simulink model "lab4_test2"  (R2016b)
settings: Solver=VariableStepAuto  StartTime=0.0  StopTime=totaltime  RelTol=1e-3
undefined symbols (not defined in the file or in its folder): h, st
libraries: xbsIndex_r4 x885
(part 1 of 2)
settings Model: Creator=rm101  LastModifiedBy=rm101

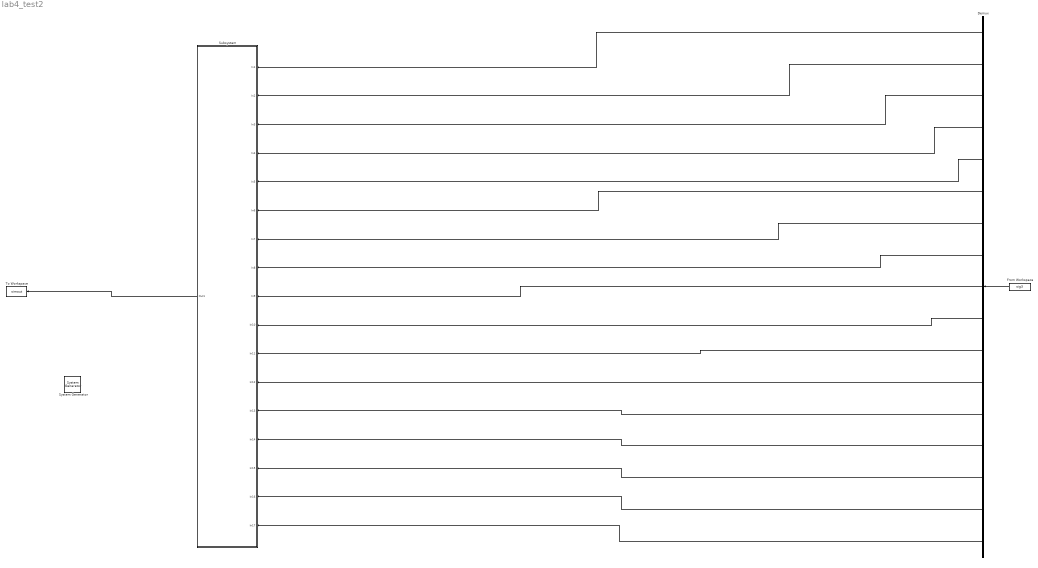
== system lab4_test2 ==
  " System Generator" : xbsIndex_r4/ System Generator  Tag=genX  xilinxfamily=zynq  part=xc7z020  speed=-1  package=clg484  synthesis_tool=Vivado  clock_wrapper=Clock Enables  directory=C:/Users/rm101/Desktop/YG/Lab4_Matlab/gen  proj_type=Vivado  Synth_file=Vivado Synthesis Defaults  Impl_file=Vivado Implementation Defaults  testbench=off  simulink_period=st  sysclk_period=st*10e8  dcm_input_clock_period=10  incr_netlist=off  trim_vbits=Everywhere in SubSystem  dbl_ovrd=According to Block Masks  core_generation=According to Block Masks  run_coregen=off  deprecated_control=off  eval_field=0  block_type=sysgen
  Demux : Demux  Outputs=17
  From Workspace : FromWorkspace  VariableName=sig3  SampleTime=0  Interpolate=off  OutputAfterFinalValue=Holding final value
  Subsystem : Subsystem
  To Workspace : ToWorkspace  VariableName=simout  SaveFormat=Timeseries  SampleTime=-1
  wires:
  From Workspace/1 -> Demux/1
  Demux/1 -> Subsystem/1(In1)
  Demux/2 -> Subsystem/2(In2)
  Demux/3 -> Subsystem/3(In3)
  Demux/4 -> Subsystem/4(In4)
  Demux/5 -> Subsystem/5(In5)
  Demux/6 -> Subsystem/6(In6)
  Demux/7 -> Subsystem/7(In7)
  Demux/8 -> Subsystem/8(In8)
  Demux/9 -> Subsystem/9(In9)
  Demux/10 -> Subsystem/10(In10)
  Demux/11 -> Subsystem/11(In11)
  Demux/12 -> Subsystem/12(In12)
  Demux/13 -> Subsystem/13(In13)
  Demux/14 -> Subsystem/14(In14)
  Demux/15 -> Subsystem/15(In15)
  Demux/16 -> Subsystem/16(In16)
  Demux/17 -> Subsystem/17(In17)
  Subsystem/1(Out1) -> To Workspace/1

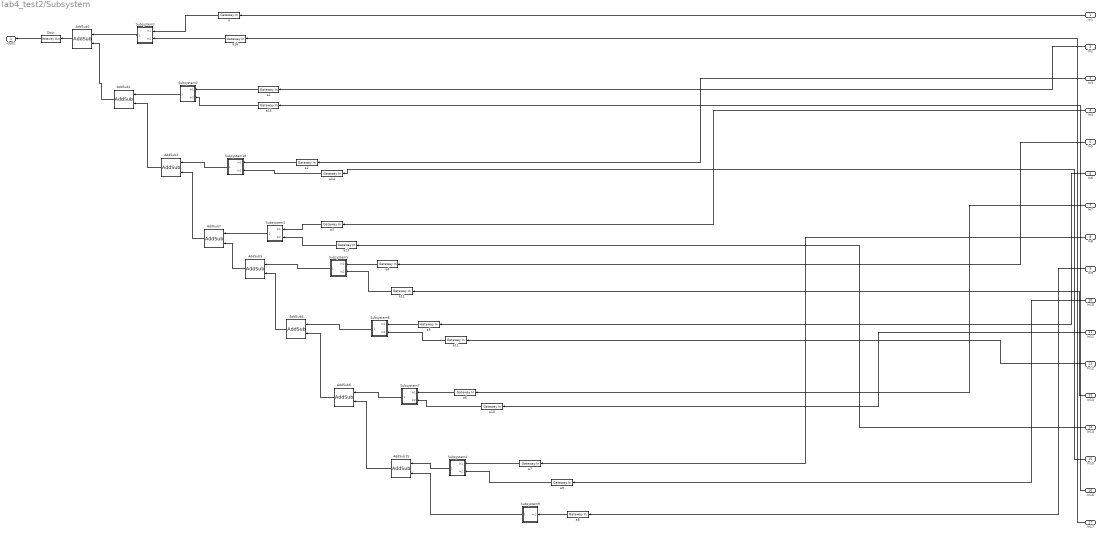
== system lab4_test2/Subsystem ==
  In1 : Inport
  In2 : Inport  Port=2
  In3 : Inport  Port=3
  In4 : Inport  Port=4
  In5 : Inport  Port=5
  In6 : Inport  Port=6
  In7 : Inport  Port=7
  In8 : Inport  Port=8
  In9 : Inport  Port=9
  In10 : Inport  Port=10
  In11 : Inport  Port=11
  In12 : Inport  Port=12
  In13 : Inport  Port=13
  In14 : Inport  Port=14
  In15 : Inport  Port=15
  In16 : Inport  Port=16
  In17 : Inport  Port=17
  AddSub{1..7,15} (8 alike) : xbsIndex_r4/AddSub  mode=Addition  use_carryin=off  use_carryout=off  en=off  latency=0  precision=User Defined  arith_type="Signed  (2's comp)"  n_bits=17  bin_pt=14  quantization=Truncate  overflow=Wrap  use_behavioral_HDL=off  hw_selection=Fabric  pipelined=off  dbl_ovrd=off  block_type=addsub
  Dout : xbsIndex_r4/Gateway Out  inherit_from_input=off  hdl_port=on  rows=1  columns=1  UseAsDAC=off  DACChannel='1'  interface=None  automatic_assignment=on  address_offset=hex2dec('00')  intf_name=''  intf_description=''  timing_constraint=None  locs_specified=off  LOCs={}  io_standard={}  block_type=gatewayout
  Subsystem1 : Subsystem
  Subsystem18 : Subsystem
  Subsystem2 : Subsystem
  Subsystem3 : Subsystem
  Subsystem4 : Subsystem
  Subsystem5 : Subsystem
  Subsystem6 : Subsystem
  Subsystem7 : Subsystem
  Subsystem9 : Subsystem
  a{,1..16} (17 alike) : xbsIndex_r4/Gateway In  gui_display_data_type=Fixed-point  arith_type="Signed  (2's comp)"  n_bits=8  bin_pt=6  preci_type=Single  exp_width=8  frac_width=24  rows=1  columns=1  quantization="Round  (unbiased: +/- Inf)"  overflow=Saturate  period=st  UseAsADC=off  ADCChannel='1'  interface=None  automatic_assignment=on  address_offset=hex2dec('00')  intf_name=''  intf_description=''  default_value=0  timing_constraint=None  locs_specified=off  LOCs={}  io_standard={}  inherit_from_input=off  hdl_port=on  dbl_ovrd=off  block_type=gatewayin
  Out1 : Outport
  wires:
  a10/1 -> Subsystem7/2(In2)
  a12/1 -> Subsystem5/2(In2)
  a11/1 -> Subsystem6/2(In2)
  a13/1 -> Subsystem3/2(In2)
  a9/1 -> Subsystem4/2(In2)
  Dout/1 -> Out1/1
  AddSub2/1 -> Dout/1
  Subsystem1/1(Out1) -> AddSub2/1
  AddSub1/1 -> AddSub2/2
  Subsystem2/1(Out1) -> AddSub1/1
  AddSub3/1 -> AddSub1/2
  Subsystem18/1(Out1) -> AddSub3/1
  AddSub7/1 -> AddSub3/2
  AddSub5/1 -> AddSub7/2
  Subsystem5/1(Out1) -> AddSub5/1
  AddSub4/1 -> AddSub5/2
  Subsystem6/1(Out1) -> AddSub4/1
  AddSub6/1 -> AddSub4/2
  Subsystem7/1(Out1) -> AddSub6/1
  AddSub15/1 -> AddSub6/2
  Subsystem3/1(Out1) -> AddSub7/1
  Subsystem4/1(Out1) -> AddSub15/1
  Subsystem9/1(Out1) -> AddSub15/2
  In2/1 -> a1/1
  In3/1 -> a2/1
  In4/1 -> a3/1
  In5/1 -> a4/1
  In6/1 -> a5/1
  In7/1 -> a6/1
  In8/1 -> a7/1
  In9/1 -> a8/1
  In10/1 -> a9/1
  In11/1 -> a10/1
  In12/1 -> a11/1
  In13/1 -> a12/1
  In14/1 -> a13/1
  In15/1 -> a14/1
  In16/1 -> a15/1
  In17/1 -> a16/1
  In1/1 -> a/1
  a/1 -> Subsystem1/1(In1)
  a1/1 -> Subsystem2/1(In1)
  a3/1 -> Subsystem3/1(In1)
  a2/1 -> Subsystem18/1(In1)
  a4/1 -> Subsystem5/1(In1)
  a5/1 -> Subsystem6/1(In1)
  a6/1 -> Subsystem7/1(In1)
  a7/1 -> Subsystem4/1(In1)
  a8/1 -> Subsystem9/1(In1)
  a14/1 -> Subsystem18/2(In2)
  a16/1 -> Subsystem1/2(In2)
  a15/1 -> Subsystem2/2(In2)

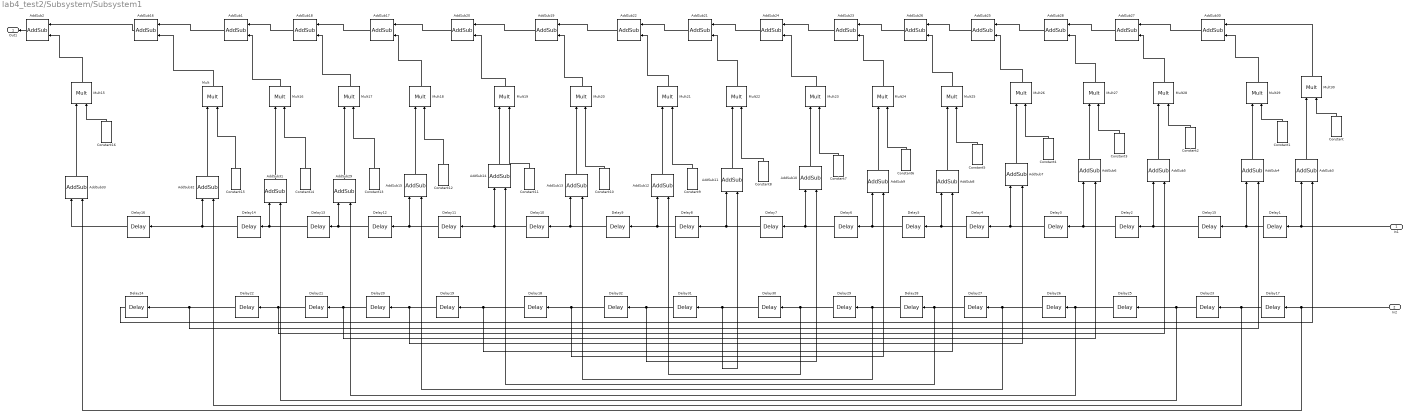
== system lab4_test2/Subsystem/Subsystem1 ==
  In1 : Inport
  In2 : Inport  Port=2
  AddSub{1..33} (33 alike) : xbsIndex_r4/AddSub  mode=Addition  use_carryin=off  use_carryout=off  en=off  latency=0  precision=User Defined  arith_type="Signed  (2's comp)"  n_bits=W  bin_pt=B  quantization=Truncate  overflow=Wrap  use_behavioral_HDL=off  hw_selection=Fabric  pipelined=off  dbl_ovrd=off  block_type=addsub
  Constant : xbsIndex_r4/Constant  const=h(1,17)  gui_display_data_type=Fixed-point  arith_type=Signed (2's comp)  n_bits=W  bin_pt=B  preci_type=Single  exp_width=8  frac_width=24  explicit_period=off  period=1  equ=P=C  opselect=C  inp2=PCIN>>17  opr=+  inp1=P  carry=CIN  dbl_ovrd=off  block_type=constant
  Constant1 : xbsIndex_r4/Constant  const=h(2,17)  gui_display_data_type=Fixed-point  arith_type=Signed (2's comp)  n_bits=W  bin_pt=B  preci_type=Single  exp_width=8  frac_width=24  explicit_period=off  period=1  equ=P=C  opselect=C  inp2=PCIN>>17  opr=+  inp1=P  carry=CIN  dbl_ovrd=off  block_type=constant
  Constant10 : xbsIndex_r4/Constant  const=h(11,17)  gui_display_data_type=Fixed-point  arith_type=Signed (2's comp)  n_bits=W  bin_pt=B  preci_type=Single  exp_width=8  frac_width=24  explicit_period=off  period=1  equ=P=C  opselect=C  inp2=PCIN>>17  opr=+  inp1=P  carry=CIN  dbl_ovrd=off  block_type=constant
  Constant11 : xbsIndex_r4/Constant  const=h(12,17)  gui_display_data_type=Fixed-point  arith_type=Signed (2's comp)  n_bits=W  bin_pt=B  preci_type=Single  exp_width=8  frac_width=24  explicit_period=off  period=1  equ=P=C  opselect=C  inp2=PCIN>>17  opr=+  inp1=P  carry=CIN  dbl_ovrd=off  block_type=constant
  Constant12 : xbsIndex_r4/Constant  const=h(13,17)  gui_display_data_type=Fixed-point  arith_type=Signed (2's comp)  n_bits=W  bin_pt=B  preci_type=Single  exp_width=8  frac_width=24  explicit_period=off  period=1  equ=P=C  opselect=C  inp2=PCIN>>17  opr=+  inp1=P  carry=CIN  dbl_ovrd=off  block_type=constant
  Constant13 : xbsIndex_r4/Constant  const=h(14,17)  gui_display_data_type=Fixed-point  arith_type=Signed (2's comp)  n_bits=W  bin_pt=B  preci_type=Single  exp_width=8  frac_width=24  explicit_period=off  period=1  equ=P=C  opselect=C  inp2=PCIN>>17  opr=+  inp1=P  carry=CIN  dbl_ovrd=off  block_type=constant
  Constant14 : xbsIndex_r4/Constant  const=h(15,17)  gui_display_data_type=Fixed-point  arith_type=Signed (2's comp)  n_bits=W  bin_pt=B  preci_type=Single  exp_width=8  frac_width=24  explicit_period=off  period=1  equ=P=C  opselect=C  inp2=PCIN>>17  opr=+  inp1=P  carry=CIN  dbl_ovrd=off  block_type=constant
  Constant15 : xbsIndex_r4/Constant  const=h(16,17)  gui_display_data_type=Fixed-point  arith_type=Signed (2's comp)  n_bits=W  bin_pt=B  preci_type=Single  exp_width=8  frac_width=24  explicit_period=off  period=1  equ=P=C  opselect=C  inp2=PCIN>>17  opr=+  inp1=P  carry=CIN  dbl_ovrd=off  block_type=constant
  Constant16 : xbsIndex_r4/Constant  const=h(17,17)  gui_display_data_type=Fixed-point  arith_type=Signed (2's comp)  n_bits=W  bin_pt=B  preci_type=Single  exp_width=8  frac_width=24  explicit_period=off  period=1  equ=P=C  opselect=C  inp2=PCIN>>17  opr=+  inp1=P  carry=CIN  dbl_ovrd=off  block_type=constant
  Constant2 : xbsIndex_r4/Constant  const=h(3,17)  gui_display_data_type=Fixed-point  arith_type=Signed (2's comp)  n_bits=W  bin_pt=B  preci_type=Single  exp_width=8  frac_width=24  explicit_period=off  period=1  equ=P=C  opselect=C  inp2=PCIN>>17  opr=+  inp1=P  carry=CIN  dbl_ovrd=off  block_type=constant
  Constant3 : xbsIndex_r4/Constant  const=h(4,17)  gui_display_data_type=Fixed-point  arith_type=Signed (2's comp)  n_bits=W  bin_pt=B  preci_type=Single  exp_width=8  frac_width=24  explicit_period=off  period=1  equ=P=C  opselect=C  inp2=PCIN>>17  opr=+  inp1=P  carry=CIN  dbl_ovrd=off  block_type=constant
  Constant4 : xbsIndex_r4/Constant  const=h(5,17)  gui_display_data_type=Fixed-point  arith_type=Signed (2's comp)  n_bits=W  bin_pt=B  preci_type=Single  exp_width=8  frac_width=24  explicit_period=off  period=1  equ=P=C  opselect=C  inp2=PCIN>>17  opr=+  inp1=P  carry=CIN  dbl_ovrd=off  block_type=constant
  Constant5 : xbsIndex_r4/Constant  const=h(6,17)  gui_display_data_type=Fixed-point  arith_type=Signed (2's comp)  n_bits=W  bin_pt=B  preci_type=Single  exp_width=8  frac_width=24  explicit_period=off  period=1  equ=P=C  opselect=C  inp2=PCIN>>17  opr=+  inp1=P  carry=CIN  dbl_ovrd=off  block_type=constant
  Constant6 : xbsIndex_r4/Constant  const=h(7,17)  gui_display_data_type=Fixed-point  arith_type=Signed (2's comp)  n_bits=W  bin_pt=B  preci_type=Single  exp_width=8  frac_width=24  explicit_period=off  period=1  equ=P=C  opselect=C  inp2=PCIN>>17  opr=+  inp1=P  carry=CIN  dbl_ovrd=off  block_type=constant
  Constant7 : xbsIndex_r4/Constant  const=h(8,17)  gui_display_data_type=Fixed-point  arith_type=Signed (2's comp)  n_bits=W  bin_pt=B  preci_type=Single  exp_width=8  frac_width=24  explicit_period=off  period=1  equ=P=C  opselect=C  inp2=PCIN>>17  opr=+  inp1=P  carry=CIN  dbl_ovrd=off  block_type=constant
  Constant8 : xbsIndex_r4/Constant  const=h(9,17)  gui_display_data_type=Fixed-point  arith_type=Signed (2's comp)  n_bits=W  bin_pt=B  preci_type=Single  exp_width=8  frac_width=24  explicit_period=off  period=1  equ=P=C  opselect=C  inp2=PCIN>>17  opr=+  inp1=P  carry=CIN  dbl_ovrd=off  block_type=constant
  Constant9 : xbsIndex_r4/Constant  const=h(10,17)  gui_display_data_type=Fixed-point  arith_type=Signed (2's comp)  n_bits=W  bin_pt=B  preci_type=Single  exp_width=8  frac_width=24  explicit_period=off  period=1  equ=P=C  opselect=C  inp2=PCIN>>17  opr=+  inp1=P  carry=CIN  dbl_ovrd=off  block_type=constant
  Delay{1..32} (32 alike) : xbsIndex_r4/Delay  rst=off  infoeditControl=Selection of Reset will increase slice count due to use of real FFs and instead of SRLs  en=off  latency=1  reg_retiming=off  dbl_ovrd=off  block_type=delay
  Mult{,15..30} (17 alike) : xbsIndex_r4/Mult  precision=User Defined  arith_type="Signed  (2's comp)"  n_bits=W  bin_pt=B  quantization="Round  (unbiased: +/- Inf)"  overflow=Flag as error  en=off  latency=0  use_behavioral_HDL=off  opt=Speed  use_embedded=on  optimum_pipeline=off  pipeline=on  dbl_ovrd=off  use_rpm=on  placement_style=Triangular  block_type=mult
  Out1 : Outport
  wires:
  AddSub2/1 -> Out1/1
  Constant14/1 -> Mult16/2
  Mult/1 -> AddSub16/2
  Mult16/1 -> AddSub1/2
  Constant15/1 -> Mult/2
  Constant13/1 -> Mult17/2
  Mult17/1 -> AddSub18/2
  Constant12/1 -> Mult18/2
  Constant11/1 -> Mult19/2
  Mult19/1 -> AddSub20/2
  Constant10/1 -> Mult20/2
  Mult20/1 -> AddSub19/2
  Constant9/1 -> Mult21/2
  Mult21/1 -> AddSub22/2
  Constant8/1 -> Mult22/2
  Constant7/1 -> Mult23/2
  Mult23/1 -> AddSub24/2
  Constant6/1 -> Mult24/2
  Constant5/1 -> Mult25/2
  Mult25/1 -> AddSub26/2
  Constant4/1 -> Mult26/2
  Mult26/1 -> AddSub25/2
  Constant3/1 -> Mult27/2
  Mult27/1 -> AddSub28/2
  Constant2/1 -> Mult28/2
  Constant1/1 -> Mult29/2
  Mult29/1 -> AddSub30/2
  Constant/1 -> Mult30/2
  AddSub1/1 -> AddSub16/1
  AddSub18/1 -> AddSub1/1
  AddSub17/1 -> AddSub18/1
  AddSub19/1 -> AddSub20/1
  AddSub22/1 -> AddSub19/1
  AddSub21/1 -> AddSub22/1
  AddSub23/1 -> AddSub24/1
  AddSub25/1 -> AddSub26/1
  AddSub28/1 -> AddSub25/1
  AddSub27/1 -> AddSub28/1
  Mult30/1 -> AddSub30/1
  Constant16/1 -> Mult15/2
  Mult15/1 -> AddSub2/2
  AddSub16/1 -> AddSub2/1
  AddSub20/1 -> AddSub17/1
  Mult18/1 -> AddSub17/2
  AddSub24/1 -> AddSub21/1
  Mult22/1 -> AddSub21/2
  AddSub26/1 -> AddSub23/1
  Mult24/1 -> AddSub23/2
  AddSub30/1 -> AddSub27/1
  Mult28/1 -> AddSub27/2
  In1/1 -> AddSub3/1, Delay1/1
  Delay1/1 -> AddSub4/1, Delay15/1
  Delay15/1 -> AddSub5/1, Delay2/1
  Delay2/1 -> AddSub6/1, Delay3/1
  Delay3/1 -> AddSub7/1, Delay4/1
  Delay4/1 -> AddSub8/1, Delay5/1
  Delay5/1 -> AddSub9/1, Delay6/1
  Delay6/1 -> AddSub10/1, Delay7/1
  Delay7/1 -> AddSub11/1, Delay8/1
  Delay8/1 -> AddSub12/1, Delay9/1
  Delay9/1 -> AddSub13/1, Delay10/1
  Delay10/1 -> AddSub14/1, Delay11/1
  Delay11/1 -> AddSub15/1, Delay12/1
  Delay12/1 -> AddSub29/1, Delay13/1
  Delay13/1 -> AddSub31/1, Delay14/1
  Delay14/1 -> AddSub32/1, Delay16/1
  In2/1 -> AddSub33/2, Delay17/1
  Delay17/1 -> AddSub32/2, Delay23/1
  Delay23/1 -> AddSub31/2, Delay25/1
  Delay25/1 -> AddSub29/2, Delay26/1
  Delay26/1 -> AddSub15/2, Delay27/1
  Delay27/1 -> AddSub14/2, Delay28/1
  Delay28/1 -> AddSub13/2, Delay29/1
  Delay29/1 -> AddSub12/2, Delay30/1
  Delay30/1 -> AddSub11/2, Delay31/1
  Delay31/1 -> AddSub10/2, Delay32/1
  Delay32/1 -> AddSub9/2, Delay18/1
  Delay18/1 -> AddSub8/2, Delay19/1
  Delay19/1 -> AddSub7/2, Delay20/1
  Delay20/1 -> AddSub6/2, Delay21/1
  Delay21/1 -> AddSub5/2, Delay22/1
  Delay22/1 -> AddSub4/2, Delay24/1
  AddSub3/1 -> Mult30/1
  Delay16/1 -> AddSub33/1
  AddSub33/1 -> Mult15/1
  AddSub32/1 -> Mult/1
  AddSub31/1 -> Mult16/1
  AddSub29/1 -> Mult17/1
  AddSub15/1 -> Mult18/1
  AddSub14/1 -> Mult19/1
  AddSub13/1 -> Mult20/1
  AddSub12/1 -> Mult21/1
  AddSub11/1 -> Mult22/1
  AddSub10/1 -> Mult23/1
  AddSub9/1 -> Mult24/1
  AddSub8/1 -> Mult25/1
  AddSub7/1 -> Mult26/1
  AddSub6/1 -> Mult27/1
  AddSub5/1 -> Mult28/1
  AddSub4/1 -> Mult29/1
  Delay24/1 -> AddSub3/2

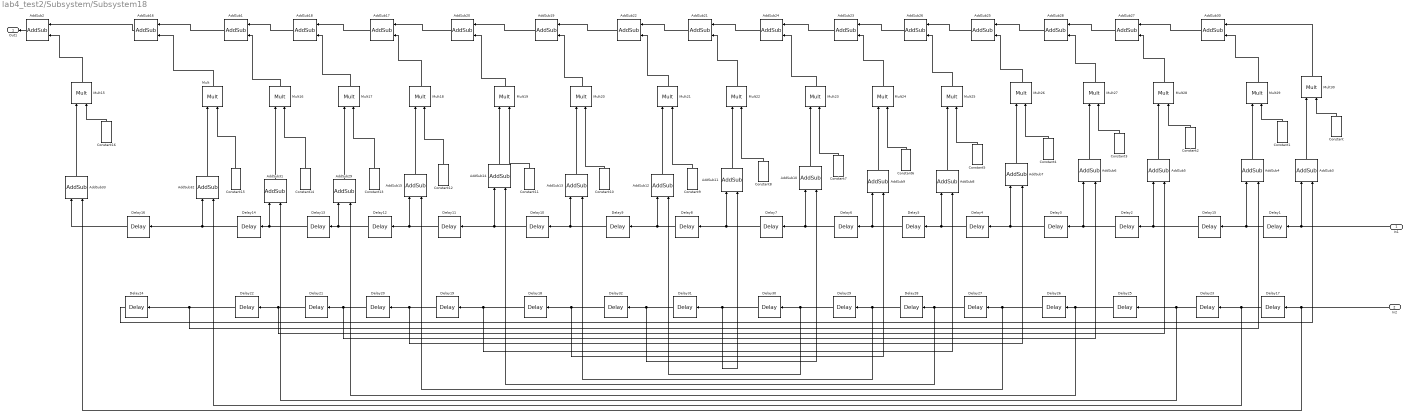
== system lab4_test2/Subsystem/Subsystem18 ==
  In1 : Inport
  In2 : Inport  Port=2
  AddSub{1..33} (33 alike) : xbsIndex_r4/AddSub  mode=Addition  use_carryin=off  use_carryout=off  en=off  latency=0  precision=User Defined  arith_type="Signed  (2's comp)"  n_bits=W  bin_pt=B  quantization=Truncate  overflow=Wrap  use_behavioral_HDL=off  hw_selection=Fabric  pipelined=off  dbl_ovrd=off  block_type=addsub
  Constant : xbsIndex_r4/Constant  const=h(1,15)  gui_display_data_type=Fixed-point  arith_type=Signed (2's comp)  n_bits=W  bin_pt=B  preci_type=Single  exp_width=8  frac_width=24  explicit_period=off  period=1  equ=P=C  opselect=C  inp2=PCIN>>17  opr=+  inp1=P  carry=CIN  dbl_ovrd=off  block_type=constant
  Constant1 : xbsIndex_r4/Constant  const=h(2,15)  gui_display_data_type=Fixed-point  arith_type=Signed (2's comp)  n_bits=W  bin_pt=B  preci_type=Single  exp_width=8  frac_width=24  explicit_period=off  period=1  equ=P=C  opselect=C  inp2=PCIN>>17  opr=+  inp1=P  carry=CIN  dbl_ovrd=off  block_type=constant
  Constant10 : xbsIndex_r4/Constant  const=h(11,15)  gui_display_data_type=Fixed-point  arith_type=Signed (2's comp)  n_bits=W  bin_pt=B  preci_type=Single  exp_width=8  frac_width=24  explicit_period=off  period=1  equ=P=C  opselect=C  inp2=PCIN>>17  opr=+  inp1=P  carry=CIN  dbl_ovrd=off  block_type=constant
  Constant11 : xbsIndex_r4/Constant  const=h(12,15)  gui_display_data_type=Fixed-point  arith_type=Signed (2's comp)  n_bits=W  bin_pt=B  preci_type=Single  exp_width=8  frac_width=24  explicit_period=off  period=1  equ=P=C  opselect=C  inp2=PCIN>>17  opr=+  inp1=P  carry=CIN  dbl_ovrd=off  block_type=constant
  Constant12 : xbsIndex_r4/Constant  const=h(13,15)  gui_display_data_type=Fixed-point  arith_type=Signed (2's comp)  n_bits=W  bin_pt=B  preci_type=Single  exp_width=8  frac_width=24  explicit_period=off  period=1  equ=P=C  opselect=C  inp2=PCIN>>17  opr=+  inp1=P  carry=CIN  dbl_ovrd=off  block_type=constant
  Constant13 : xbsIndex_r4/Constant  const=h(14,15)  gui_display_data_type=Fixed-point  arith_type=Signed (2's comp)  n_bits=W  bin_pt=B  preci_type=Single  exp_width=8  frac_width=24  explicit_period=off  period=1  equ=P=C  opselect=C  inp2=PCIN>>17  opr=+  inp1=P  carry=CIN  dbl_ovrd=off  block_type=constant
  Constant14 : xbsIndex_r4/Constant  const=h(15,15)  gui_display_data_type=Fixed-point  arith_type=Signed (2's comp)  n_bits=W  bin_pt=B  preci_type=Single  exp_width=8  frac_width=24  explicit_period=off  period=1  equ=P=C  opselect=C  inp2=PCIN>>17  opr=+  inp1=P  carry=CIN  dbl_ovrd=off  block_type=constant
  Constant15 : xbsIndex_r4/Constant  const=h(16,15)  gui_display_data_type=Fixed-point  arith_type=Signed (2's comp)  n_bits=W  bin_pt=B  preci_type=Single  exp_width=8  frac_width=24  explicit_period=off  period=1  equ=P=C  opselect=C  inp2=PCIN>>17  opr=+  inp1=P  carry=CIN  dbl_ovrd=off  block_type=constant
  Constant16 : xbsIndex_r4/Constant  const=h(17,15)  gui_display_data_type=Fixed-point  arith_type=Signed (2's comp)  n_bits=W  bin_pt=B  preci_type=Single  exp_width=8  frac_width=24  explicit_period=off  period=1  equ=P=C  opselect=C  inp2=PCIN>>17  opr=+  inp1=P  carry=CIN  dbl_ovrd=off  block_type=constant
  Constant2 : xbsIndex_r4/Constant  const=h(3,15)  gui_display_data_type=Fixed-point  arith_type=Signed (2's comp)  n_bits=W  bin_pt=B  preci_type=Single  exp_width=8  frac_width=24  explicit_period=off  period=1  equ=P=C  opselect=C  inp2=PCIN>>17  opr=+  inp1=P  carry=CIN  dbl_ovrd=off  block_type=constant
  Constant3 : xbsIndex_r4/Constant  const=h(4,15)  gui_display_data_type=Fixed-point  arith_type=Signed (2's comp)  n_bits=W  bin_pt=B  preci_type=Single  exp_width=8  frac_width=24  explicit_period=off  period=1  equ=P=C  opselect=C  inp2=PCIN>>17  opr=+  inp1=P  carry=CIN  dbl_ovrd=off  block_type=constant
  Constant4 : xbsIndex_r4/Constant  const=h(5,15)  gui_display_data_type=Fixed-point  arith_type=Signed (2's comp)  n_bits=W  bin_pt=B  preci_type=Single  exp_width=8  frac_width=24  explicit_period=off  period=1  equ=P=C  opselect=C  inp2=PCIN>>17  opr=+  inp1=P  carry=CIN  dbl_ovrd=off  block_type=constant
  Constant5 : xbsIndex_r4/Constant  const=h(6,15)  gui_display_data_type=Fixed-point  arith_type=Signed (2's comp)  n_bits=W  bin_pt=B  preci_type=Single  exp_width=8  frac_width=24  explicit_period=off  period=1  equ=P=C  opselect=C  inp2=PCIN>>17  opr=+  inp1=P  carry=CIN  dbl_ovrd=off  block_type=constant
  Constant6 : xbsIndex_r4/Constant  const=h(7,15)  gui_display_data_type=Fixed-point  arith_type=Signed (2's comp)  n_bits=W  bin_pt=B  preci_type=Single  exp_width=8  frac_width=24  explicit_period=off  period=1  equ=P=C  opselect=C  inp2=PCIN>>17  opr=+  inp1=P  carry=CIN  dbl_ovrd=off  block_type=constant
  Constant7 : xbsIndex_r4/Constant  const=h(8,15)  gui_display_data_type=Fixed-point  arith_type=Signed (2's comp)  n_bits=W  bin_pt=B  preci_type=Single  exp_width=8  frac_width=24  explicit_period=off  period=1  equ=P=C  opselect=C  inp2=PCIN>>17  opr=+  inp1=P  carry=CIN  dbl_ovrd=off  block_type=constant
  Constant8 : xbsIndex_r4/Constant  const=h(9,15)  gui_display_data_type=Fixed-point  arith_type=Signed (2's comp)  n_bits=W  bin_pt=B  preci_type=Single  exp_width=8  frac_width=24  explicit_period=off  period=1  equ=P=C  opselect=C  inp2=PCIN>>17  opr=+  inp1=P  carry=CIN  dbl_ovrd=off  block_type=constant
  Constant9 : xbsIndex_r4/Constant  const=h(10,15)  gui_display_data_type=Fixed-point  arith_type=Signed (2's comp)  n_bits=W  bin_pt=B  preci_type=Single  exp_width=8  frac_width=24  explicit_period=off  period=1  equ=P=C  opselect=C  inp2=PCIN>>17  opr=+  inp1=P  carry=CIN  dbl_ovrd=off  block_type=constant
  Delay{1..32} (32 alike) : xbsIndex_r4/Delay  rst=off  infoeditControl=Selection of Reset will increase slice count due to use of real FFs and instead of SRLs  en=off  latency=1  reg_retiming=off  dbl_ovrd=off  block_type=delay
  Mult{,15..30} (17 alike) : xbsIndex_r4/Mult  precision=User Defined  arith_type="Signed  (2's comp)"  n_bits=W  bin_pt=B  quantization="Round  (unbiased: +/- Inf)"  overflow=Flag as error  en=off  latency=0  use_behavioral_HDL=off  opt=Speed  use_embedded=on  optimum_pipeline=off  pipeline=on  dbl_ovrd=off  use_rpm=on  placement_style=Triangular  block_type=mult
  Out1 : Outport
  wires:
  AddSub2/1 -> Out1/1
  Constant14/1 -> Mult16/2
  Mult/1 -> AddSub16/2
  Mult16/1 -> AddSub1/2
  Constant15/1 -> Mult/2
  Constant13/1 -> Mult17/2
  Mult17/1 -> AddSub18/2
  Constant12/1 -> Mult18/2
  Constant11/1 -> Mult19/2
  Mult19/1 -> AddSub20/2
  Constant10/1 -> Mult20/2
  Mult20/1 -> AddSub19/2
  Constant9/1 -> Mult21/2
  Mult21/1 -> AddSub22/2
  Constant8/1 -> Mult22/2
  Constant7/1 -> Mult23/2
  Mult23/1 -> AddSub24/2
  Constant6/1 -> Mult24/2
  Constant5/1 -> Mult25/2
  Mult25/1 -> AddSub26/2
  Constant4/1 -> Mult26/2
  Mult26/1 -> AddSub25/2
  Constant3/1 -> Mult27/2
  Mult27/1 -> AddSub28/2
  Constant2/1 -> Mult28/2
  Constant1/1 -> Mult29/2
  Mult29/1 -> AddSub30/2
  Constant/1 -> Mult30/2
  AddSub1/1 -> AddSub16/1
  AddSub18/1 -> AddSub1/1
  AddSub17/1 -> AddSub18/1
  AddSub19/1 -> AddSub20/1
  AddSub22/1 -> AddSub19/1
  AddSub21/1 -> AddSub22/1
  AddSub23/1 -> AddSub24/1
  AddSub25/1 -> AddSub26/1
  AddSub28/1 -> AddSub25/1
  AddSub27/1 -> AddSub28/1
  Mult30/1 -> AddSub30/1
  Constant16/1 -> Mult15/2
  Mult15/1 -> AddSub2/2
  AddSub16/1 -> AddSub2/1
  AddSub20/1 -> AddSub17/1
  Mult18/1 -> AddSub17/2
  AddSub24/1 -> AddSub21/1
  Mult22/1 -> AddSub21/2
  AddSub26/1 -> AddSub23/1
  Mult24/1 -> AddSub23/2
  AddSub30/1 -> AddSub27/1
  Mult28/1 -> AddSub27/2
  In1/1 -> AddSub3/1, Delay1/1
  Delay1/1 -> AddSub4/1, Delay15/1
  Delay15/1 -> AddSub5/1, Delay2/1
  Delay2/1 -> AddSub6/1, Delay3/1
  Delay3/1 -> AddSub7/1, Delay4/1
  Delay4/1 -> AddSub8/1, Delay5/1
  Delay5/1 -> AddSub9/1, Delay6/1
  Delay6/1 -> AddSub10/1, Delay7/1
  Delay7/1 -> AddSub11/1, Delay8/1
  Delay8/1 -> AddSub12/1, Delay9/1
  Delay9/1 -> AddSub13/1, Delay10/1
  Delay10/1 -> AddSub14/1, Delay11/1
  Delay11/1 -> AddSub15/1, Delay12/1
  Delay12/1 -> AddSub29/1, Delay13/1
  Delay13/1 -> AddSub31/1, Delay14/1
  Delay14/1 -> AddSub32/1, Delay16/1
  In2/1 -> AddSub33/2, Delay17/1
  Delay17/1 -> AddSub32/2, Delay23/1
  Delay23/1 -> AddSub31/2, Delay25/1
  Delay25/1 -> AddSub29/2, Delay26/1
  Delay26/1 -> AddSub15/2, Delay27/1
  Delay27/1 -> AddSub14/2, Delay28/1
  Delay28/1 -> AddSub13/2, Delay29/1
  Delay29/1 -> AddSub12/2, Delay30/1
  Delay30/1 -> AddSub11/2, Delay31/1
  Delay31/1 -> AddSub10/2, Delay32/1
  Delay32/1 -> AddSub9/2, Delay18/1
  Delay18/1 -> AddSub8/2, Delay19/1
  Delay19/1 -> AddSub7/2, Delay20/1
  Delay20/1 -> AddSub6/2, Delay21/1
  Delay21/1 -> AddSub5/2, Delay22/1
  Delay22/1 -> AddSub4/2, Delay24/1
  AddSub3/1 -> Mult30/1
  Delay16/1 -> AddSub33/1
  AddSub33/1 -> Mult15/1
  AddSub32/1 -> Mult/1
  AddSub31/1 -> Mult16/1
  AddSub29/1 -> Mult17/1
  AddSub15/1 -> Mult18/1
  AddSub14/1 -> Mult19/1
  AddSub13/1 -> Mult20/1
  AddSub12/1 -> Mult21/1
  AddSub11/1 -> Mult22/1
  AddSub10/1 -> Mult23/1
  AddSub9/1 -> Mult24/1
  AddSub8/1 -> Mult25/1
  AddSub7/1 -> Mult26/1
  AddSub6/1 -> Mult27/1
  AddSub5/1 -> Mult28/1
  AddSub4/1 -> Mult29/1
  Delay24/1 -> AddSub3/2

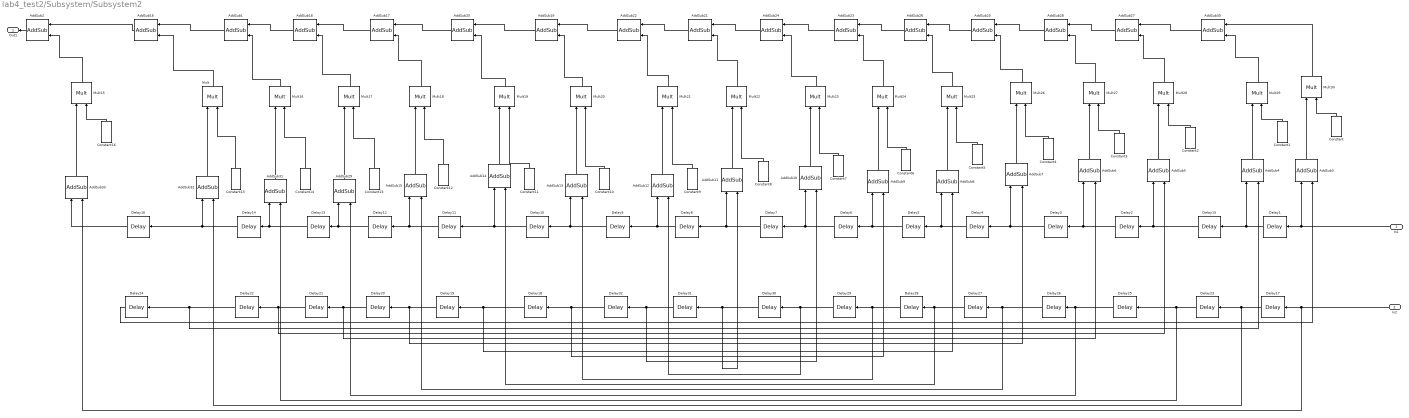
== system lab4_test2/Subsystem/Subsystem2 ==
  In1 : Inport
  In2 : Inport  Port=2
  AddSub{1..33} (33 alike) : xbsIndex_r4/AddSub  mode=Addition  use_carryin=off  use_carryout=off  en=off  latency=0  precision=User Defined  arith_type="Signed  (2's comp)"  n_bits=W  bin_pt=B  quantization=Truncate  overflow=Wrap  use_behavioral_HDL=off  hw_selection=Fabric  pipelined=off  dbl_ovrd=off  block_type=addsub
  Constant : xbsIndex_r4/Constant  const=h(1,16)  gui_display_data_type=Fixed-point  arith_type=Signed (2's comp)  n_bits=W  bin_pt=B  preci_type=Single  exp_width=8  frac_width=24  explicit_period=off  period=1  equ=P=C  opselect=C  inp2=PCIN>>17  opr=+  inp1=P  carry=CIN  dbl_ovrd=off  block_type=constant
  Constant1 : xbsIndex_r4/Constant  const=h(2,16)  gui_display_data_type=Fixed-point  arith_type=Signed (2's comp)  n_bits=W  bin_pt=B  preci_type=Single  exp_width=8  frac_width=24  explicit_period=off  period=1  equ=P=C  opselect=C  inp2=PCIN>>17  opr=+  inp1=P  carry=CIN  dbl_ovrd=off  block_type=constant
  Constant10 : xbsIndex_r4/Constant  const=h(11,16)  gui_display_data_type=Fixed-point  arith_type=Signed (2's comp)  n_bits=W  bin_pt=B  preci_type=Single  exp_width=8  frac_width=24  explicit_period=off  period=1  equ=P=C  opselect=C  inp2=PCIN>>17  opr=+  inp1=P  carry=CIN  dbl_ovrd=off  block_type=constant
  Constant11 : xbsIndex_r4/Constant  const=h(12,16)  gui_display_data_type=Fixed-point  arith_type=Signed (2's comp)  n_bits=W  bin_pt=B  preci_type=Single  exp_width=8  frac_width=24  explicit_period=off  period=1  equ=P=C  opselect=C  inp2=PCIN>>17  opr=+  inp1=P  carry=CIN  dbl_ovrd=off  block_type=constant
  Constant12 : xbsIndex_r4/Constant  const=h(13,16)  gui_display_data_type=Fixed-point  arith_type=Signed (2's comp)  n_bits=W  bin_pt=B  preci_type=Single  exp_width=8  frac_width=24  explicit_period=off  period=1  equ=P=C  opselect=C  inp2=PCIN>>17  opr=+  inp1=P  carry=CIN  dbl_ovrd=off  block_type=constant
  Constant13 : xbsIndex_r4/Constant  const=h(14,16)  gui_display_data_type=Fixed-point  arith_type=Signed (2's comp)  n_bits=W  bin_pt=B  preci_type=Single  exp_width=8  frac_width=24  explicit_period=off  period=1  equ=P=C  opselect=C  inp2=PCIN>>17  opr=+  inp1=P  carry=CIN  dbl_ovrd=off  block_type=constant
  Constant14 : xbsIndex_r4/Constant  const=h(15,16)  gui_display_data_type=Fixed-point  arith_type=Signed (2's comp)  n_bits=W  bin_pt=B  preci_type=Single  exp_width=8  frac_width=24  explicit_period=off  period=1  equ=P=C  opselect=C  inp2=PCIN>>17  opr=+  inp1=P  carry=CIN  dbl_ovrd=off  block_type=constant
  Constant15 : xbsIndex_r4/Constant  const=h(16,16)  gui_display_data_type=Fixed-point  arith_type=Signed (2's comp)  n_bits=W  bin_pt=B  preci_type=Single  exp_width=8  frac_width=24  explicit_period=off  period=1  equ=P=C  opselect=C  inp2=PCIN>>17  opr=+  inp1=P  carry=CIN  dbl_ovrd=off  block_type=constant
  Constant16 : xbsIndex_r4/Constant  const=h(17,16)  gui_display_data_type=Fixed-point  arith_type=Signed (2's comp)  n_bits=W  bin_pt=B  preci_type=Single  exp_width=8  frac_width=24  explicit_period=off  period=1  equ=P=C  opselect=C  inp2=PCIN>>17  opr=+  inp1=P  carry=CIN  dbl_ovrd=off  block_type=constant
  Constant2 : xbsIndex_r4/Constant  const=h(3,16)  gui_display_data_type=Fixed-point  arith_type=Signed (2's comp)  n_bits=W  bin_pt=B  preci_type=Single  exp_width=8  frac_width=24  explicit_period=off  period=1  equ=P=C  opselect=C  inp2=PCIN>>17  opr=+  inp1=P  carry=CIN  dbl_ovrd=off  block_type=constant
  Constant3 : xbsIndex_r4/Constant  const=h(4,16)  gui_display_data_type=Fixed-point  arith_type=Signed (2's comp)  n_bits=W  bin_pt=B  preci_type=Single  exp_width=8  frac_width=24  explicit_period=off  period=1  equ=P=C  opselect=C  inp2=PCIN>>17  opr=+  inp1=P  carry=CIN  dbl_ovrd=off  block_type=constant
  Constant4 : xbsIndex_r4/Constant  const=h(5,16)  gui_display_data_type=Fixed-point  arith_type=Signed (2's comp)  n_bits=W  bin_pt=B  preci_type=Single  exp_width=8  frac_width=24  explicit_period=off  period=1  equ=P=C  opselect=C  inp2=PCIN>>17  opr=+  inp1=P  carry=CIN  dbl_ovrd=off  block_type=constant
  Constant5 : xbsIndex_r4/Constant  const=h(6,16)  gui_display_data_type=Fixed-point  arith_type=Signed (2's comp)  n_bits=W  bin_pt=B  preci_type=Single  exp_width=8  frac_width=24  explicit_period=off  period=1  equ=P=C  opselect=C  inp2=PCIN>>17  opr=+  inp1=P  carry=CIN  dbl_ovrd=off  block_type=constant
  Constant6 : xbsIndex_r4/Constant  const=h(7,16)  gui_display_data_type=Fixed-point  arith_type=Signed (2's comp)  n_bits=W  bin_pt=B  preci_type=Single  exp_width=8  frac_width=24  explicit_period=off  period=1  equ=P=C  opselect=C  inp2=PCIN>>17  opr=+  inp1=P  carry=CIN  dbl_ovrd=off  block_type=constant
  Constant7 : xbsIndex_r4/Constant  const=h(8,16)  gui_display_data_type=Fixed-point  arith_type=Signed (2's comp)  n_bits=W  bin_pt=B  preci_type=Single  exp_width=8  frac_width=24  explicit_period=off  period=1  equ=P=C  opselect=C  inp2=PCIN>>17  opr=+  inp1=P  carry=CIN  dbl_ovrd=off  block_type=constant
  Constant8 : xbsIndex_r4/Constant  const=h(9,16)  gui_display_data_type=Fixed-point  arith_type=Signed (2's comp)  n_bits=W  bin_pt=B  preci_type=Single  exp_width=8  frac_width=24  explicit_period=off  period=1  equ=P=C  opselect=C  inp2=PCIN>>17  opr=+  inp1=P  carry=CIN  dbl_ovrd=off  block_type=constant
  Constant9 : xbsIndex_r4/Constant  const=h(10,16)  gui_display_data_type=Fixed-point  arith_type=Signed (2's comp)  n_bits=W  bin_pt=B  preci_type=Single  exp_width=8  frac_width=24  explicit_period=off  period=1  equ=P=C  opselect=C  inp2=PCIN>>17  opr=+  inp1=P  carry=CIN  dbl_ovrd=off  block_type=constant
  Delay{1..32} (32 alike) : xbsIndex_r4/Delay  rst=off  infoeditControl=Selection of Reset will increase slice count due to use of real FFs and instead of SRLs  en=off  latency=1  reg_retiming=off  dbl_ovrd=off  block_type=delay
  Mult{,15..30} (17 alike) : xbsIndex_r4/Mult  precision=User Defined  arith_type="Signed  (2's comp)"  n_bits=W  bin_pt=B  quantization="Round  (unbiased: +/- Inf)"  overflow=Flag as error  en=off  latency=0  use_behavioral_HDL=off  opt=Speed  use_embedded=on  optimum_pipeline=off  pipeline=on  dbl_ovrd=off  use_rpm=on  placement_style=Triangular  block_type=mult
  Out1 : Outport
  wires:
  AddSub2/1 -> Out1/1
  Constant14/1 -> Mult16/2
  Mult/1 -> AddSub16/2
  Mult16/1 -> AddSub1/2
  Constant15/1 -> Mult/2
  Constant13/1 -> Mult17/2
  Mult17/1 -> AddSub18/2
  Constant12/1 -> Mult18/2
  Constant11/1 -> Mult19/2
  Mult19/1 -> AddSub20/2
  Constant10/1 -> Mult20/2
  Mult20/1 -> AddSub19/2
  Constant9/1 -> Mult21/2
  Mult21/1 -> AddSub22/2
  Constant8/1 -> Mult22/2
  Constant7/1 -> Mult23/2
  Mult23/1 -> AddSub24/2
  Constant6/1 -> Mult24/2
  Constant5/1 -> Mult25/2
  Mult25/1 -> AddSub26/2
  Constant4/1 -> Mult26/2
  Mult26/1 -> AddSub25/2
  Constant3/1 -> Mult27/2
  Mult27/1 -> AddSub28/2
  Constant2/1 -> Mult28/2
  Constant1/1 -> Mult29/2
  Mult29/1 -> AddSub30/2
  Constant/1 -> Mult30/2
  AddSub1/1 -> AddSub16/1
  AddSub18/1 -> AddSub1/1
  AddSub17/1 -> AddSub18/1
  AddSub19/1 -> AddSub20/1
  AddSub22/1 -> AddSub19/1
  AddSub21/1 -> AddSub22/1
  AddSub23/1 -> AddSub24/1
  AddSub25/1 -> AddSub26/1
  AddSub28/1 -> AddSub25/1
  AddSub27/1 -> AddSub28/1
  Mult30/1 -> AddSub30/1
  Constant16/1 -> Mult15/2
  Mult15/1 -> AddSub2/2
  AddSub16/1 -> AddSub2/1
  AddSub20/1 -> AddSub17/1
  Mult18/1 -> AddSub17/2
  AddSub24/1 -> AddSub21/1
  Mult22/1 -> AddSub21/2
  AddSub26/1 -> AddSub23/1
  Mult24/1 -> AddSub23/2
  AddSub30/1 -> AddSub27/1
  Mult28/1 -> AddSub27/2
  In1/1 -> AddSub3/1, Delay1/1
  Delay1/1 -> AddSub4/1, Delay15/1
  Delay15/1 -> AddSub5/1, Delay2/1
  Delay2/1 -> AddSub6/1, Delay3/1
  Delay3/1 -> AddSub7/1, Delay4/1
  Delay4/1 -> AddSub8/1, Delay5/1
  Delay5/1 -> AddSub9/1, Delay6/1
  Delay6/1 -> AddSub10/1, Delay7/1
  Delay7/1 -> AddSub11/1, Delay8/1
  Delay8/1 -> AddSub12/1, Delay9/1
  Delay9/1 -> AddSub13/1, Delay10/1
  Delay10/1 -> AddSub14/1, Delay11/1
  Delay11/1 -> AddSub15/1, Delay12/1
  Delay12/1 -> AddSub29/1, Delay13/1
  Delay13/1 -> AddSub31/1, Delay14/1
  Delay14/1 -> AddSub32/1, Delay16/1
  In2/1 -> AddSub33/2, Delay17/1
  Delay17/1 -> AddSub32/2, Delay23/1
  Delay23/1 -> AddSub31/2, Delay25/1
  Delay25/1 -> AddSub29/2, Delay26/1
  Delay26/1 -> AddSub15/2, Delay27/1
  Delay27/1 -> AddSub14/2, Delay28/1
  Delay28/1 -> AddSub13/2, Delay29/1
  Delay29/1 -> AddSub12/2, Delay30/1
  Delay30/1 -> AddSub11/2, Delay31/1
  Delay31/1 -> AddSub10/2, Delay32/1
  Delay32/1 -> AddSub9/2, Delay18/1
  Delay18/1 -> AddSub8/2, Delay19/1
  Delay19/1 -> AddSub7/2, Delay20/1
  Delay20/1 -> AddSub6/2, Delay21/1
  Delay21/1 -> AddSub5/2, Delay22/1
  Delay22/1 -> AddSub4/2, Delay24/1
  AddSub3/1 -> Mult30/1
  Delay16/1 -> AddSub33/1
  AddSub33/1 -> Mult15/1
  AddSub32/1 -> Mult/1
  AddSub31/1 -> Mult16/1
  AddSub29/1 -> Mult17/1
  AddSub15/1 -> Mult18/1
  AddSub14/1 -> Mult19/1
  AddSub13/1 -> Mult20/1
  AddSub12/1 -> Mult21/1
  AddSub11/1 -> Mult22/1
  AddSub10/1 -> Mult23/1
  AddSub9/1 -> Mult24/1
  AddSub8/1 -> Mult25/1
  AddSub7/1 -> Mult26/1
  AddSub6/1 -> Mult27/1
  AddSub5/1 -> Mult28/1
  AddSub4/1 -> Mult29/1
  Delay24/1 -> AddSub3/2

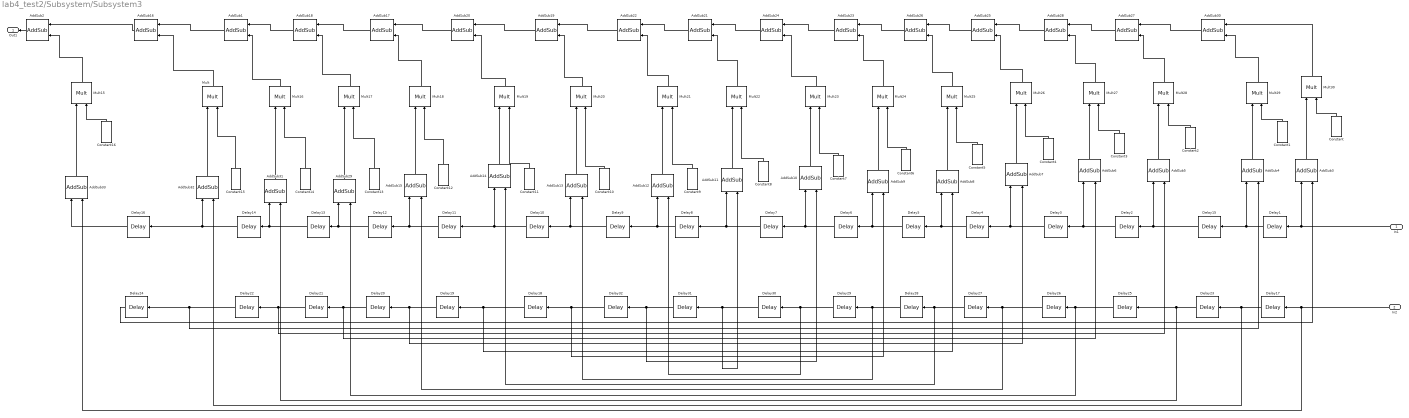
== system lab4_test2/Subsystem/Subsystem3 ==
  In1 : Inport
  In2 : Inport  Port=2
  AddSub{1..33} (33 alike) : xbsIndex_r4/AddSub  mode=Addition  use_carryin=off  use_carryout=off  en=off  latency=0  precision=User Defined  arith_type="Signed  (2's comp)"  n_bits=W  bin_pt=B  quantization=Truncate  overflow=Wrap  use_behavioral_HDL=off  hw_selection=Fabric  pipelined=off  dbl_ovrd=off  block_type=addsub
  Constant : xbsIndex_r4/Constant  const=h(1,14)  gui_display_data_type=Fixed-point  arith_type=Signed (2's comp)  n_bits=W  bin_pt=B  preci_type=Single  exp_width=8  frac_width=24  explicit_period=off  period=1  equ=P=C  opselect=C  inp2=PCIN>>17  opr=+  inp1=P  carry=CIN  dbl_ovrd=off  block_type=constant
  Constant1 : xbsIndex_r4/Constant  const=h(2,14)  gui_display_data_type=Fixed-point  arith_type=Signed (2's comp)  n_bits=W  bin_pt=B  preci_type=Single  exp_width=8  frac_width=24  explicit_period=off  period=1  equ=P=C  opselect=C  inp2=PCIN>>17  opr=+  inp1=P  carry=CIN  dbl_ovrd=off  block_type=constant
  Constant10 : xbsIndex_r4/Constant  const=h(11,14)  gui_display_data_type=Fixed-point  arith_type=Signed (2's comp)  n_bits=W  bin_pt=B  preci_type=Single  exp_width=8  frac_width=24  explicit_period=off  period=1  equ=P=C  opselect=C  inp2=PCIN>>17  opr=+  inp1=P  carry=CIN  dbl_ovrd=off  block_type=constant
  Constant11 : xbsIndex_r4/Constant  const=h(12,14)  gui_display_data_type=Fixed-point  arith_type=Signed (2's comp)  n_bits=W  bin_pt=B  preci_type=Single  exp_width=8  frac_width=24  explicit_period=off  period=1  equ=P=C  opselect=C  inp2=PCIN>>17  opr=+  inp1=P  carry=CIN  dbl_ovrd=off  block_type=constant
  Constant12 : xbsIndex_r4/Constant  const=h(13,14)  gui_display_data_type=Fixed-point  arith_type=Signed (2's comp)  n_bits=W  bin_pt=B  preci_type=Single  exp_width=8  frac_width=24  explicit_period=off  period=1  equ=P=C  opselect=C  inp2=PCIN>>17  opr=+  inp1=P  carry=CIN  dbl_ovrd=off  block_type=constant
  Constant13 : xbsIndex_r4/Constant  const=h(14,14)  gui_display_data_type=Fixed-point  arith_type=Signed (2's comp)  n_bits=W  bin_pt=B  preci_type=Single  exp_width=8  frac_width=24  explicit_period=off  period=1  equ=P=C  opselect=C  inp2=PCIN>>17  opr=+  inp1=P  carry=CIN  dbl_ovrd=off  block_type=constant
  Constant14 : xbsIndex_r4/Constant  const=h(15,14)  gui_display_data_type=Fixed-point  arith_type=Signed (2's comp)  n_bits=W  bin_pt=B  preci_type=Single  exp_width=8  frac_width=24  explicit_period=off  period=1  equ=P=C  opselect=C  inp2=PCIN>>17  opr=+  inp1=P  carry=CIN  dbl_ovrd=off  block_type=constant
  Constant15 : xbsIndex_r4/Constant  const=h(16,14)  gui_display_data_type=Fixed-point  arith_type=Signed (2's comp)  n_bits=W  bin_pt=B  preci_type=Single  exp_width=8  frac_width=24  explicit_period=off  period=1  equ=P=C  opselect=C  inp2=PCIN>>17  opr=+  inp1=P  carry=CIN  dbl_ovrd=off  block_type=constant
  Constant16 : xbsIndex_r4/Constant  const=h(17,14)  gui_display_data_type=Fixed-point  arith_type=Signed (2's comp)  n_bits=W  bin_pt=B  preci_type=Single  exp_width=8  frac_width=24  explicit_period=off  period=1  equ=P=C  opselect=C  inp2=PCIN>>17  opr=+  inp1=P  carry=CIN  dbl_ovrd=off  block_type=constant
  Constant2 : xbsIndex_r4/Constant  const=h(3,14)  gui_display_data_type=Fixed-point  arith_type=Signed (2's comp)  n_bits=W  bin_pt=B  preci_type=Single  exp_width=8  frac_width=24  explicit_period=off  period=1  equ=P=C  opselect=C  inp2=PCIN>>17  opr=+  inp1=P  carry=CIN  dbl_ovrd=off  block_type=constant
  Constant3 : xbsIndex_r4/Constant  const=h(4,14)  gui_display_data_type=Fixed-point  arith_type=Signed (2's comp)  n_bits=W  bin_pt=B  preci_type=Single  exp_width=8  frac_width=24  explicit_period=off  period=1  equ=P=C  opselect=C  inp2=PCIN>>17  opr=+  inp1=P  carry=CIN  dbl_ovrd=off  block_type=constant
  Constant4 : xbsIndex_r4/Constant  const=h(5,14)  gui_display_data_type=Fixed-point  arith_type=Signed (2's comp)  n_bits=W  bin_pt=B  preci_type=Single  exp_width=8  frac_width=24  explicit_period=off  period=1  equ=P=C  opselect=C  inp2=PCIN>>17  opr=+  inp1=P  carry=CIN  dbl_ovrd=off  block_type=constant
  Constant5 : xbsIndex_r4/Constant  const=h(6,14)  gui_display_data_type=Fixed-point  arith_type=Signed (2's comp)  n_bits=W  bin_pt=B  preci_type=Single  exp_width=8  frac_width=24  explicit_period=off  period=1  equ=P=C  opselect=C  inp2=PCIN>>17  opr=+  inp1=P  carry=CIN  dbl_ovrd=off  block_type=constant
  Constant6 : xbsIndex_r4/Constant  const=h(7,14)  gui_display_data_type=Fixed-point  arith_type=Signed (2's comp)  n_bits=W  bin_pt=B  preci_type=Single  exp_width=8  frac_width=24  explicit_period=off  period=1  equ=P=C  opselect=C  inp2=PCIN>>17  opr=+  inp1=P  carry=CIN  dbl_ovrd=off  block_type=constant
  Constant7 : xbsIndex_r4/Constant  const=h(8,14)  gui_display_data_type=Fixed-point  arith_type=Signed (2's comp)  n_bits=W  bin_pt=B  preci_type=Single  exp_width=8  frac_width=24  explicit_period=off  period=1  equ=P=C  opselect=C  inp2=PCIN>>17  opr=+  inp1=P  carry=CIN  dbl_ovrd=off  block_type=constant
  Constant8 : xbsIndex_r4/Constant  const=h(9,14)  gui_display_data_type=Fixed-point  arith_type=Signed (2's comp)  n_bits=W  bin_pt=B  preci_type=Single  exp_width=8  frac_width=24  explicit_period=off  period=1  equ=P=C  opselect=C  inp2=PCIN>>17  opr=+  inp1=P  carry=CIN  dbl_ovrd=off  block_type=constant
  Constant9 : xbsIndex_r4/Constant  const=h(10,14)  gui_display_data_type=Fixed-point  arith_type=Signed (2's comp)  n_bits=W  bin_pt=B  preci_type=Single  exp_width=8  frac_width=24  explicit_period=off  period=1  equ=P=C  opselect=C  inp2=PCIN>>17  opr=+  inp1=P  carry=CIN  dbl_ovrd=off  block_type=constant
  Delay{1..32} (32 alike) : xbsIndex_r4/Delay  rst=off  infoeditControl=Selection of Reset will increase slice count due to use of real FFs and instead of SRLs  en=off  latency=1  reg_retiming=off  dbl_ovrd=off  block_type=delay
  Mult{,15..30} (17 alike) : xbsIndex_r4/Mult  precision=User Defined  arith_type="Signed  (2's comp)"  n_bits=W  bin_pt=B  quantization="Round  (unbiased: +/- Inf)"  overflow=Flag as error  en=off  latency=0  use_behavioral_HDL=off  opt=Speed  use_embedded=on  optimum_pipeline=off  pipeline=on  dbl_ovrd=off  use_rpm=on  placement_style=Triangular  block_type=mult
  Out1 : Outport
  wires:
  AddSub2/1 -> Out1/1
  Constant14/1 -> Mult16/2
  Mult/1 -> AddSub16/2
  Mult16/1 -> AddSub1/2
  Constant15/1 -> Mult/2
  Constant13/1 -> Mult17/2
  Mult17/1 -> AddSub18/2
  Constant12/1 -> Mult18/2
  Constant11/1 -> Mult19/2
  Mult19/1 -> AddSub20/2
  Constant10/1 -> Mult20/2
  Mult20/1 -> AddSub19/2
  Constant9/1 -> Mult21/2
  Mult21/1 -> AddSub22/2
  Constant8/1 -> Mult22/2
  Constant7/1 -> Mult23/2
  Mult23/1 -> AddSub24/2
  Constant6/1 -> Mult24/2
  Constant5/1 -> Mult25/2
  Mult25/1 -> AddSub26/2
  Constant4/1 -> Mult26/2
  Mult26/1 -> AddSub25/2
  Constant3/1 -> Mult27/2
  Mult27/1 -> AddSub28/2
  Constant2/1 -> Mult28/2
  Constant1/1 -> Mult29/2
  Mult29/1 -> AddSub30/2
  Constant/1 -> Mult30/2
  AddSub1/1 -> AddSub16/1
  AddSub18/1 -> AddSub1/1
  AddSub17/1 -> AddSub18/1
  AddSub19/1 -> AddSub20/1
  AddSub22/1 -> AddSub19/1
  AddSub21/1 -> AddSub22/1
  AddSub23/1 -> AddSub24/1
  AddSub25/1 -> AddSub26/1
  AddSub28/1 -> AddSub25/1
  AddSub27/1 -> AddSub28/1
  Mult30/1 -> AddSub30/1
  Constant16/1 -> Mult15/2
  Mult15/1 -> AddSub2/2
  AddSub16/1 -> AddSub2/1
  AddSub20/1 -> AddSub17/1
  Mult18/1 -> AddSub17/2
  AddSub24/1 -> AddSub21/1
  Mult22/1 -> AddSub21/2
  AddSub26/1 -> AddSub23/1
  Mult24/1 -> AddSub23/2
  AddSub30/1 -> AddSub27/1
  Mult28/1 -> AddSub27/2
  In1/1 -> AddSub3/1, Delay1/1
  Delay1/1 -> AddSub4/1, Delay15/1
  Delay15/1 -> AddSub5/1, Delay2/1
  Delay2/1 -> AddSub6/1, Delay3/1
  Delay3/1 -> AddSub7/1, Delay4/1
  Delay4/1 -> AddSub8/1, Delay5/1
  Delay5/1 -> AddSub9/1, Delay6/1
  Delay6/1 -> AddSub10/1, Delay7/1
  Delay7/1 -> AddSub11/1, Delay8/1
  Delay8/1 -> AddSub12/1, Delay9/1
  Delay9/1 -> AddSub13/1, Delay10/1
  Delay10/1 -> AddSub14/1, Delay11/1
  Delay11/1 -> AddSub15/1, Delay12/1
  Delay12/1 -> AddSub29/1, Delay13/1
  Delay13/1 -> AddSub31/1, Delay14/1
  Delay14/1 -> AddSub32/1, Delay16/1
  In2/1 -> AddSub33/2, Delay17/1
  Delay17/1 -> AddSub32/2, Delay23/1
  Delay23/1 -> AddSub31/2, Delay25/1
  Delay25/1 -> AddSub29/2, Delay26/1
  Delay26/1 -> AddSub15/2, Delay27/1
  Delay27/1 -> AddSub14/2, Delay28/1
  Delay28/1 -> AddSub13/2, Delay29/1
  Delay29/1 -> AddSub12/2, Delay30/1
  Delay30/1 -> AddSub11/2, Delay31/1
  Delay31/1 -> AddSub10/2, Delay32/1
  Delay32/1 -> AddSub9/2, Delay18/1
  Delay18/1 -> AddSub8/2, Delay19/1
  Delay19/1 -> AddSub7/2, Delay20/1
  Delay20/1 -> AddSub6/2, Delay21/1
  Delay21/1 -> AddSub5/2, Delay22/1
  Delay22/1 -> AddSub4/2, Delay24/1
  AddSub3/1 -> Mult30/1
  Delay16/1 -> AddSub33/1
  AddSub33/1 -> Mult15/1
  AddSub32/1 -> Mult/1
  AddSub31/1 -> Mult16/1
  AddSub29/1 -> Mult17/1
  AddSub15/1 -> Mult18/1
  AddSub14/1 -> Mult19/1
  AddSub13/1 -> Mult20/1
  AddSub12/1 -> Mult21/1
  AddSub11/1 -> Mult22/1
  AddSub10/1 -> Mult23/1
  AddSub9/1 -> Mult24/1
  AddSub8/1 -> Mult25/1
  AddSub7/1 -> Mult26/1
  AddSub6/1 -> Mult27/1
  AddSub5/1 -> Mult28/1
  AddSub4/1 -> Mult29/1
  Delay24/1 -> AddSub3/2
